simulink model "SIMU_FONCTIONNEL_2021"  (R2021a)
settings: Solver=VariableStepAuto  StartTime=0.0  StopTime=10  RelTol=1e-3
model workspace (MAT data in the model file):
  R = 3.18
  kfcm = 0.0109
libraries: pid_lib x2
settings Model: Creator=nada2516  LastModifiedBy=elisa

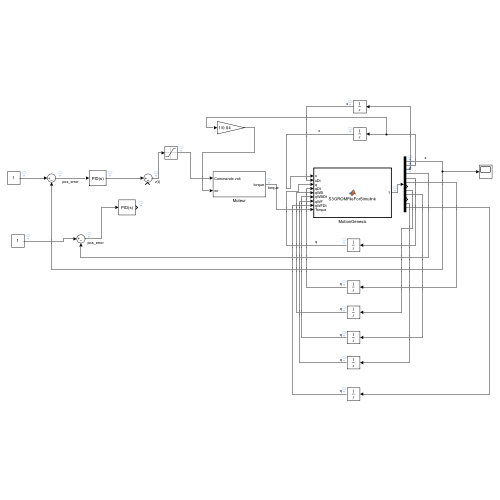
[thumbnail: Simulink's stored preview of the top-level diagram]
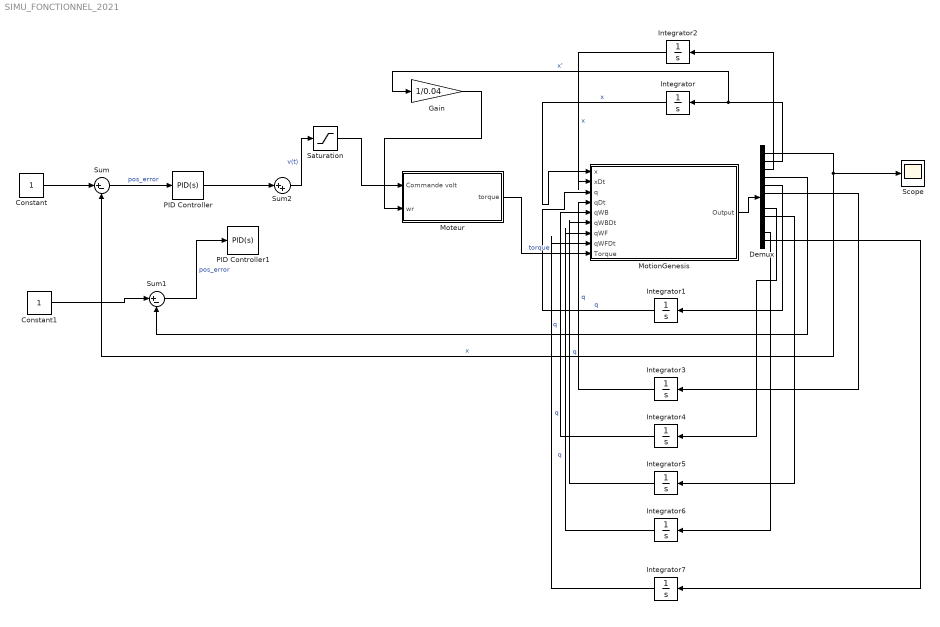
== system SIMU_FONCTIONNEL_2021 ==
  Constant : Constant
  Constant1 : Constant
  Demux : Demux  Outputs=12
  Gain : Gain  Gain=1/0.04
  Integrator{,1..7} (8 alike) : Integrator
  Moteur : Subsystem
  MotionGenesis : MATLAB Function  TreatAsAtomicUnit=on
  PID Controller : pid_lib/PID Controller  Controller=PID  Form=Parallel  TimeDomain=Continuous-time  UseExternalTs=off  SampleTime=-1  IntegratorMethod=Forward Euler  FilterMethod=Forward Euler  ControllerParametersSource=internal  P=140  I=17  D=1  N=100  UseFilter=on  TunerSelectOption=Transfer Function Based (PID Tuner App)  InitialConditionSource=internal  InitialConditionForIntegrator=0  InitialConditionForFilter=0  DifferentiatorICPrevScaledInput=0  ExternalReset=none  TrackingMode=off  Kt=1  LimitOutput=off  SatLimitsSource=internal  UpperSaturationLimit=inf  LowerSaturationLimit=-inf  LinearizeAsGain=on  AntiWindupMode=none  Kb=1  POutMin=[]  POutMax=[]  IOutMin=[]  IOutMax=[]  DOutMin=[]  DOutMax=[]  NOutMin=[]  NOutMax=[]  SumOutMin=[]  SumOutMax=[]  SaturationOutMin=[]  SaturationOutMax=[]  PParamMin=[]  PParamMax=[]  IParamMin=[]  IParamMax=[]  DParamMin=[]  DParamMax=[]  NParamMin=[]  NParamMax=[]  KbParamMin=[]  KbParamMax=[]  KtParamMin=[]  KtParamMax=[]  KbOutMin=[]  KbOutMax=[]  KtOutMin=[]  KtOutMax=[]  IntegratorOutMin=[]  IntegratorOutMax=[]  FilterOutMin=[]  FilterOutMax=[]  SumI1OutMin=[]  SumI1OutMax=[]  SumI2OutMin=[]  SumI2OutMax=[]  SumI3OutMin=[]  SumI3OutMax=[]  SumI4OutMin=[]  SumI4OutMax=[]  SumDOutMin=[]  SumDOutMax=[]  DifferentiatorOutMin=[]  DifferentiatorOutMax=[]  FilterDiffOutCoefMin=[]  FilterDiffOutCoefMax=[]  ReciprocalOutMin=[]  ReciprocalOutMax=[]  SumDenOutMin=[]  SumDenOutMax=[]  SumNumOutMin=[]  SumNumOutMax=[]  DivideOutMin=[]  DivideOutMax=[]  UdiffTsProdOutMin=[]  UdiffTsProdOutMax=[]  NTsProdOutMin=[]  NTsProdOutMax=[]  UintegralTsProdOutMin=[]  UintegralTsProdOutMax=[]  UngainTsProdOutMin=[]  UngainTsProdOutMax=[]  IntegratorContinuousStateAttributes=''  IntegratorStateMustResolveToSignalObject=off  IntegratorRTWStateStorageClass=Auto  FilterContinuousStateAttributes=''  FilterStateMustResolveToSignalObject=off  FilterRTWStateStorageClass=Auto  ParallelPVariant=InternalParameters  IdealPVariant=Disabled  IVariant=InternalParameters  DVariant=InternalParameters  IntegratorVariant=Continuous  SatVariant=Disabled  AWVariant=Passthrough  PCopyVariant=Disabled  TRVariant=Disabled  FdbkBlocksVariant=Forward  IdealPFdbkVariant=Disabled  SatFdbkVariant=Disabled  DerivativeFilterVariant=ContFilter  NVariant=InternalParameters  NCopyVariant=Disabled  FilterICVariant=InternalICsFilter  IntegratorICVariant=InternalICs  ExternalResetVariant=Disabled  TRSumVariant=Passthrough  SumFdbkVariant=Disabled  SumVariant=Sum_PID  TsampFilterVariant=InternalTs  TsampNgainVariant=Passthrough  TsampIntegralVariant=Disabled_SignalSpec  ExternalSaturationOutDataTypeStr=Inherit: Same as second input
  PID Controller1 : pid_lib/PID Controller  Controller=PID  Form=Parallel  TimeDomain=Continuous-time  UseExternalTs=off  SampleTime=-1  IntegratorMethod=Forward Euler  FilterMethod=Forward Euler  ControllerParametersSource=internal  P=1  I=1  D=1  N=100  UseFilter=on  TunerSelectOption=Transfer Function Based (PID Tuner App)  InitialConditionSource=internal  InitialConditionForIntegrator=0  InitialConditionForFilter=0  DifferentiatorICPrevScaledInput=0  ExternalReset=none  TrackingMode=off  Kt=1  LimitOutput=off  SatLimitsSource=internal  UpperSaturationLimit=inf  LowerSaturationLimit=-inf  LinearizeAsGain=on  AntiWindupMode=none  Kb=1  POutMin=[]  POutMax=[]  IOutMin=[]  IOutMax=[]  DOutMin=[]  DOutMax=[]  NOutMin=[]  NOutMax=[]  SumOutMin=[]  SumOutMax=[]  SaturationOutMin=[]  SaturationOutMax=[]  PParamMin=[]  PParamMax=[]  IParamMin=[]  IParamMax=[]  DParamMin=[]  DParamMax=[]  NParamMin=[]  NParamMax=[]  KbParamMin=[]  KbParamMax=[]  KtParamMin=[]  KtParamMax=[]  KbOutMin=[]  KbOutMax=[]  KtOutMin=[]  KtOutMax=[]  IntegratorOutMin=[]  IntegratorOutMax=[]  FilterOutMin=[]  FilterOutMax=[]  SumI1OutMin=[]  SumI1OutMax=[]  SumI2OutMin=[]  SumI2OutMax=[]  SumI3OutMin=[]  SumI3OutMax=[]  SumI4OutMin=[]  SumI4OutMax=[]  SumDOutMin=[]  SumDOutMax=[]  DifferentiatorOutMin=[]  DifferentiatorOutMax=[]  FilterDiffOutCoefMin=[]  FilterDiffOutCoefMax=[]  ReciprocalOutMin=[]  ReciprocalOutMax=[]  SumDenOutMin=[]  SumDenOutMax=[]  SumNumOutMin=[]  SumNumOutMax=[]  DivideOutMin=[]  DivideOutMax=[]  UdiffTsProdOutMin=[]  UdiffTsProdOutMax=[]  NTsProdOutMin=[]  NTsProdOutMax=[]  UintegralTsProdOutMin=[]  UintegralTsProdOutMax=[]  UngainTsProdOutMin=[]  UngainTsProdOutMax=[]  IntegratorContinuousStateAttributes=''  IntegratorStateMustResolveToSignalObject=off  IntegratorRTWStateStorageClass=Auto  FilterContinuousStateAttributes=''  FilterStateMustResolveToSignalObject=off  FilterRTWStateStorageClass=Auto  ParallelPVariant=InternalParameters  IdealPVariant=Disabled  IVariant=InternalParameters  DVariant=InternalParameters  IntegratorVariant=Continuous  SatVariant=Disabled  AWVariant=Passthrough  PCopyVariant=Disabled  TRVariant=Disabled  FdbkBlocksVariant=Forward  IdealPFdbkVariant=Disabled  SatFdbkVariant=Disabled  DerivativeFilterVariant=ContFilter  NVariant=InternalParameters  NCopyVariant=Disabled  FilterICVariant=InternalICsFilter  IntegratorICVariant=InternalICs  ExternalResetVariant=Disabled  TRSumVariant=Passthrough  SumFdbkVariant=Disabled  SumVariant=Sum_PID  TsampFilterVariant=InternalTs  TsampNgainVariant=Passthrough  TsampIntegralVariant=Disabled_SignalSpec  ExternalSaturationOutDataTypeStr=Inherit: Same as second input
  Saturation : Saturate  UpperLimit=12  LowerLimit=0
  Scope : Scope
  Sum : Sum  Inputs=|+-
  Sum1 : Sum  Inputs=|+-
  Sum2 : Sum  Inputs=|++
  wires:
  Constant/1 -> Sum/1
  Sum/1 -> PID Controller/1  "pos_error"
  PID Controller/1 -> Sum2/1
  MotionGenesis/1(Output) -> Demux/1
  Integrator/1 -> MotionGenesis/1(x)  "x"
  Integrator1/1 -> MotionGenesis/3(q)  "q"
  Demux/1 -> Sum/2, Scope/1  "x"
  Demux/2 -> Gain/1, Integrator/1  "x'"
  Demux/3 -> Integrator2/1
  Integrator2/1 -> MotionGenesis/2(xDt)  "x"
  Demux/4 -> Sum1/2
  Demux/5 -> Integrator1/1
  Demux/6 -> Integrator3/1
  Integrator3/1 -> MotionGenesis/4(qDt)  "q"
  Demux/8 -> Integrator4/1
  Integrator4/1 -> MotionGenesis/5(qWB)  "q"
  Demux/9 -> Integrator5/1
  Integrator5/1 -> MotionGenesis/6(qWBDt)  "q"
  Integrator6/1 -> MotionGenesis/7(qWF)  "q"
  Demux/11 -> Integrator6/1
  Demux/12 -> Integrator7/1
  Integrator7/1 -> MotionGenesis/8(qWFDt)  "q"
  Moteur/1(torque) -> MotionGenesis/9(Torque)  "torque"
  Gain/1 -> Moteur/2(wr)
  Constant1/1 -> Sum1/1
  Sum1/1 -> PID Controller1/1  "pos_error"
  Sum2/1 -> Saturation/1  "v(t)"
  Saturation/1 -> Moteur/1(Commande volt)

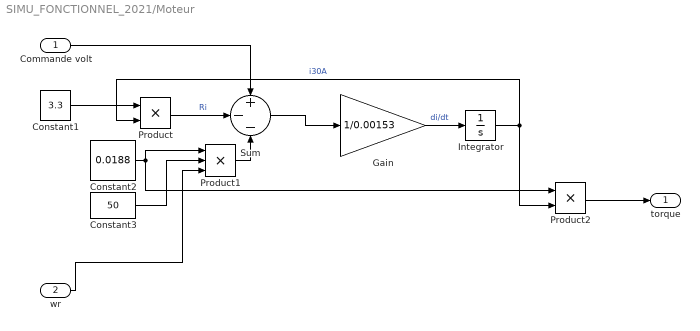
== system SIMU_FONCTIONNEL_2021/Moteur ==
  Commande volt : Inport
  wr : Inport  Port=2
  Constant1 : Constant  Value=3.3
  Constant2 : Constant  Value=0.0188
  Constant3 : Constant  Value=50
  Gain : Gain  Gain=1/0.00153
  Integrator : Integrator
  Product : Product
  Product1 : Product  Inputs=3
  Product2 : Product
  Sum : Sum  Inputs=+--
  torque : Outport
  wires:
  Integrator/1 -> Product2/2, Product/2  "i30A"
  Product/1 -> Sum/2  "Ri"
  Sum/1 -> Gain/1
  Constant3/1 -> Product1/2
  Product1/1 -> Sum/3
  Commande volt/1 -> Sum/1
  Constant2/1 -> Product2/1, Product1/1
  Gain/1 -> Integrator/1  "di/dt"
  Constant1/1 -> Product/1
  wr/1 -> Product1/3
  Product2/1 -> torque/1

== matlab function SIMU_FONCTIONNEL_2021/MotionGenesis ==
  data: Output output; x input; xDt input; q input; qDt input; qWB input; qWBDt input; qWF input; qWFDt input; Torque input
function Output  = S3GROMFileForSimulink( x, xDt, q, qDt, qWB, qWBDt, qWF, qWFDt, Torque )
if( nargin ~= 9 ) error( 'S3GROMFileForSimulink expects 9 (not %d) command line arguments.', nargin ),  end
%===========================================================================
% File: S3GROMFileForSimulink.m created Jun 20 2024 by MotionGenesis 6.3.
% Portions copyright (c) 2009-2023 Motion Genesis LLC.  Rights reserved.
% MotionGenesis Student Licensee: Elisabeth. (until February 2028).
% Paid-up MotionGenesis Student licensees are granted the right
% to distribute this code for legal student-academic (non-professional) purposes only,
% provided this copyright notice appears in all copies and distributions.
%===========================================================================
% The software is provided "as is", without warranty of any kind, express or    
% implied, including but not limited to the warranties of merchantability or    
% fitness for a particular purpose. In no event shall the authors, contributors,
% or copyright holders be liable for any claim, damages or other liability,     
% whether in an action of contract, tort, or otherwise, arising from, out of, or
% in connection with the software or the use or other dealings in the software. 
%===========================================================================


%-------------------------------+--------------------------+-------------------+-----------------
% Quantity                      | Value                    | Units             | Description
%-------------------------------|--------------------------|-------------------|-----------------
b                               =  0.3;                    % UNITS               Constant
g                               =  9.81;                   % m/s^2               Constant
L                               =  0.5;                    % m                   Constant
mB                              =  0.0018;                 % kg                  Constant
mF                              =  0.0018;                 % kg                  Constant
mP                              =  0.5;                    % kg                  Constant
mQ                              =  0.05;                   % kg                  Constant
mR                              =  3;                      % kg                  Constant
rayon                           =  0.04;                   % m                   Constant
%-------------------------------+--------------------------+-------------------+-----------------

% Unit conversions
RADtoDEG = 180.0 / pi;

%===========================================================================
qDDt = -2*(mP+2*mQ)*Torque*cos(q)/(L*rayon*(2*mB*(mP+3*mQ)+2*mF*(mP+3*mQ)+1.333333333333333*(mP+mR)*(mP+3*mQ)-mP*(mP+2*mQ)*cos(q)^2))  ...
- mP*(mP+2*mQ)*sin(q)*cos(q)*qDt^2/(2*mB*(mP+3*mQ)+2*mF*(mP+3*mQ)+1.333333333333333*(mP+mR)*(mP+3*mQ)-mP*(mP+2*mQ)*cos(q)^2)  ...
- 2*(mP+mR+1.5*mB+1.5*mF)*(g*L*(mP+2*mQ)*sin(q)+2*b*qDt)/(L^2*(2*mB*(mP+3*mQ)+2*mF*(mP+3*mQ)+1.333333333333333*(mP+mR)*(mP+3*mQ)-  ...
mP*(mP+2*mQ)*cos(q)^2));
qWBDDt = -0.6666666666666666*(2*L*(mP+3*mQ)*Torque+mP*rayon*L^2*(mP+3*mQ)*sin(q)*qDt^2+1.5*mP*rayon*cos(q)*(g*L*(mP+2*mQ)*sin(q)+  ...
2*b*qDt))/(L*rayon^2*(2*mB*(mP+3*mQ)+2*mF*(mP+3*mQ)+1.333333333333333*(mP+mR)*(mP+3*mQ)-mP*(mP+2*mQ)*cos(q)^2));
xDDt = 0.6666666666666666*(2*L*(mP+3*mQ)*Torque+mP*rayon*L^2*(mP+3*mQ)*sin(q)*qDt^2+1.5*mP*rayon*cos(q)*(g*L*(mP+2*mQ)*sin(q)+2*b*  ...
qDt))/(L*rayon*(2*mB*(mP+3*mQ)+2*mF*(mP+3*mQ)+1.333333333333333*(mP+mR)*(mP+3*mQ)-mP*(mP+2*mQ)*cos(q)^2));
qWFDDt = -0.6666666666666666*(2*L*(mP+3*mQ)*Torque+mP*rayon*L^2*(mP+3*mQ)*sin(q)*qDt^2+1.5*mP*rayon*cos(q)*(g*L*(mP+2*mQ)*sin(q)+  ...
2*b*qDt))/(L*rayon^2*(2*mB*(mP+3*mQ)+2*mF*(mP+3*mQ)+1.333333333333333*(mP+mR)*(mP+3*mQ)-mP*(mP+2*mQ)*cos(q)^2));



%===========================================================================
Output = zeros( 1, 12 );

Output(1) = x;
Output(2) = xDt;
Output(3) = xDDt;
Output(4) = q*RADtoDEG;
Output(5) = qDt*RADtoDEG;
Output(6) = qDDt*RADtoDEG;
Output(7) = qWB*RADtoDEG;
Output(8) = qWBDt*RADtoDEG;
Output(9) = qWBDDt*RADtoDEG;
Output(10) = qWF*RADtoDEG;
Output(11) = qWFDt*RADtoDEG;
Output(12) = qWFDDt*RADtoDEG;

%==============================================
end    % End of function S3GROMFileForSimulink
%==============================================
